simulink model "CustArch_v20"  (R2020a)
settings: Solver=FixedStepDiscrete  StartTime=0.0  StopTime=840000  RelTol=1e-3
libraries: simulink x84, hdlsllib x53
(part 1 of 2)
settings Model: DataTypeOverride=Off  FPTRunName=FPA_Reference  SimulationMode=accelerator  PauseTimes=5600  PacingRate=40  Creator=BuccelliLab  LastModifiedBy=diflo
settings SolverCC: AutoInsertRateTranBlk=on  MinimalZcImpactIntegration=on
settings DataIOCC: LimitDataPoints=on  SaveOutput=off  SaveTime=off  ReturnWorkspaceOutputs=off
settings OptimizationCC: BlockReduction=off  ConditionallyExecuteInputs=off  DefaultParameterBehavior=Inlined  LifeSpan=inf
settings DebuggingCC: SignalRangeChecking=warning  ReadBeforeWriteMsg=DisableAll  WriteAfterWriteMsg=DisableAll  WriteAfterReadMsg=DisableAll  AlgebraicLoopMsg=error  MultiTaskDSMMsg=none  SingleTaskRateTransMsg=error  ParameterDowncastMsg=warning  ParameterOverflowMsg=warning  AllowSymbolicDim=off  StrictBusMsg=ErrorOnBusTreatedAsVector  SFUnexpectedBacktrackingDiag=warning  SFNoUnconditionalDefaultTransitionDiag=warning  SFExecutionAtInitializationDiag=none  ArithmeticOperatorsInVariantConditions=warning
settings HardwareCC: ProdBitPerPointer=32  ProdBitPerSizeT=32  ProdBitPerPtrDiffT=32  ProdLargestAtomicFloat=None  ProdIntDivRoundTo=Undefined  ProdEndianess=Unspecified  ProdWordSize=32  ProdHWDeviceType=ASIC/FPGA->ASIC/FPGA  TargetBitPerPointer=64  TargetBitPerSizeT=64  TargetBitPerPtrDiffT=64  TargetLongLongMode=on  TargetIntDivRoundTo=Zero  TargetEndianess=LittleEndian  TargetWordSize=64  TargetHWDeviceType=Custom Processor->MATLAB Host Computer  ProdEqTarget=off
settings ModelReferenceCC: UpdateModelReferenceTargets=IfOutOfDate
settings SFSimCC: SFSimEcho=off  SimUseLocalCustomCode=off  CustomCodeUndefinedFunction=UseInterfaceOnly
settings RTWCC: RTWUseLocalCustomCode=off
settings CodeAppCC: StateflowObjectComments=on
settings GRTTargetCC: TargetLangStandard=C89/C90 (ANSI)
settings ConfigComp: CovScope=ReferencedModels  CovMetricSettings=dw  CovHtmlReporting=on  CovSaveCumulativeToWorkspaceVar=on  CovSaveSingleToWorkspaceVar=on  CovExternalEMLEnable=off  CovSFcnEnable=off

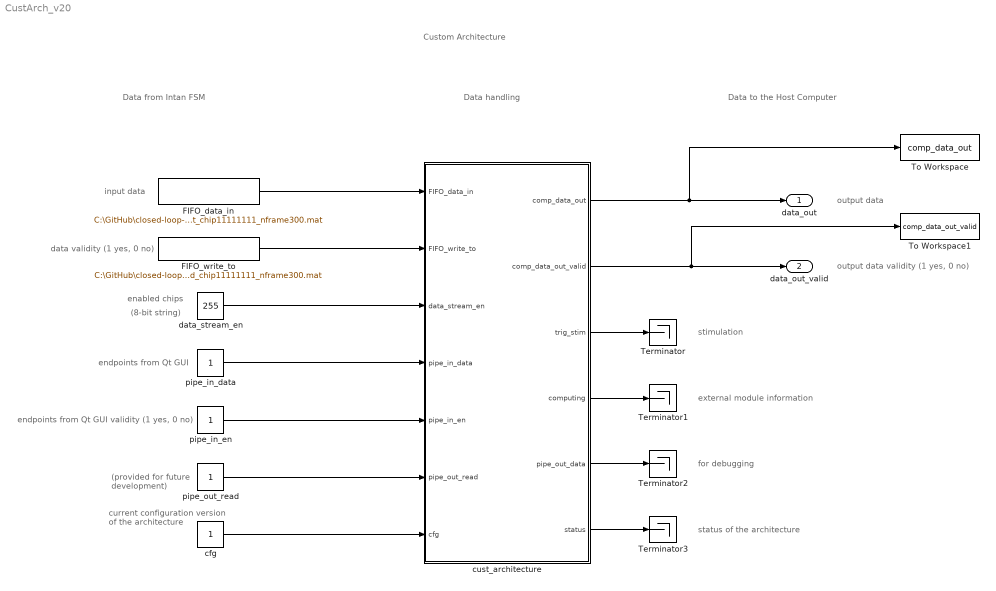
== system CustArch_v20 ==
  note: Data handling
  note: Custom Architecture
  note: output data validity (1 yes, 0 no)
  note: endpoints from Qt GUI
  note: (8-bit string)
  note: enabled chips
  note: data validity (1 yes, 0 no)
  note: input data
  note: endpoints from Qt GUI validity (1 yes, 0 no)
  note: (provided for future
      | development)
  note: current configuration
      | version of the
      | architecture
  note: output data
  note: Data to the Host Computer
  note: stimulation
  note: external module information
  note: for debugging
  note: status of the architecture
  note: Data from Intan FSM
  FIFO_data_in : FromFile  FileName=C:\GitHub\closed-loop-neuroscience\Mattia\Custom_architecture\CustArch_debug\In_Out_Simulink\In\invivo_fsm_out_chip11111111_nframe300.mat  OutDataTypeStr=uint16  SampleTime=1  ExtrapolationBeforeFirstDataPoint=Hold first value  InterpolationWithinTimeRange=Zero order hold  ExtrapolationAfterLastDataPoint=Hold last value
  FIFO_write_to : FromFile  FileName=C:\GitHub\closed-loop-neuroscience\Mattia\Custom_architecture\CustArch_debug\In_Out_Simulink\In\invivo_fsm_valid_chip11111111_nframe300.mat  OutDataTypeStr=boolean  SampleTime=1
  Terminator{,1..3} (4 alike) : Terminator
  To Workspace : ToWorkspace  VariableName=comp_data_out  SaveFormat=Timeseries  SampleTime=-1
  To Workspace1 : ToWorkspace  VariableName=comp_data_out_valid  SaveFormat=Timeseries  SampleTime=-1
  cfg : Constant  OutDataTypeStr=uint16  SampleTime=-1
  cust_architecture : Subsystem
  data_stream_en : Constant  Value=255  OutDataTypeStr=uint8  SampleTime=-1
  pipe_in_data : Constant  OutDataTypeStr=uint16  SampleTime=-1
  pipe_in_en : Constant  OutDataTypeStr=boolean  SampleTime=-1
  pipe_out_read : Constant  OutDataTypeStr=boolean  SampleTime=-1
  data_out : Outport  VectorParamsAs1DForOutWhenUnconnected=off
  data_out_valid : Outport  Port=2  VectorParamsAs1DForOutWhenUnconnected=off
  wires:
  FIFO_data_in/1 -> cust_architecture/1(FIFO_data_in)
  FIFO_write_to/1 -> cust_architecture/2(FIFO_write_to)
  cust_architecture/1(comp_data_out) -> To Workspace/1, data_out/1
  cust_architecture/2(comp_data_out_valid) -> To Workspace1/1, data_out_valid/1
  data_stream_en/1 -> cust_architecture/3(data_stream_en)
  pipe_in_data/1 -> cust_architecture/4(pipe_in_data)
  pipe_in_en/1 -> cust_architecture/5(pipe_in_en)
  pipe_out_read/1 -> cust_architecture/6(pipe_out_read)
  cfg/1 -> cust_architecture/7(cfg)
  cust_architecture/3(trig_stim) -> Terminator/1
  cust_architecture/4(computing) -> Terminator1/1
  cust_architecture/5(pipe_out_data) -> Terminator2/1
  cust_architecture/6(status) -> Terminator3/1

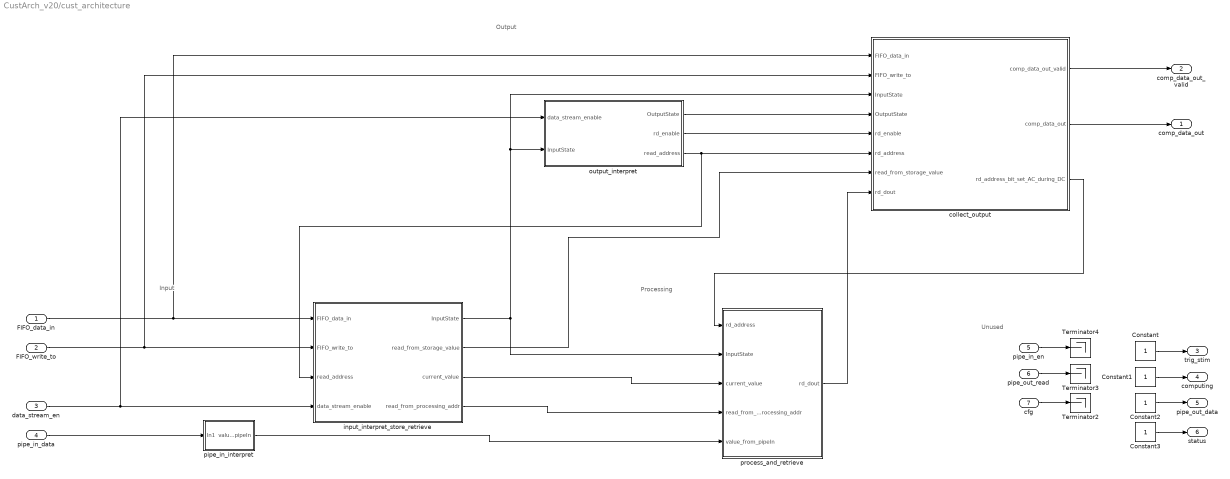
== system CustArch_v20/cust_architecture ==
  note: Unused
  note: Processing
  note: Output
  note: Input
  FIFO_data_in : Inport
  FIFO_write_to : Inport  Port=2
  data_stream_en : Inport  Port=3
  pipe_in_data : Inport  Port=4
  pipe_in_en : Inport  Port=5
  pipe_out_read : Inport  Port=6
  cfg : Inport  Port=7
  Constant : Constant  OutDataTypeStr=uint8  SampleTime=-1
  Constant1 : Constant  OutDataTypeStr=boolean  SampleTime=-1
  Constant2 : Constant  OutDataTypeStr=uint16  SampleTime=-1
  Constant3 : Constant  OutDataTypeStr=uint16  SampleTime=-1
  Terminator2 : Terminator
  Terminator3 : Terminator
  Terminator4 : Terminator
  collect_output : Subsystem
  input_interpret_store_retrieve : Subsystem
  output_interpret : Subsystem
  pipe_in_interpret : Subsystem
  process_and_retrieve : Subsystem
  comp_data_out : Outport  VectorParamsAs1DForOutWhenUnconnected=off
  comp_data_out_valid : Outport  Port=2  OutDataTypeStr=boolean  VectorParamsAs1DForOutWhenUnconnected=off
  trig_stim : Outport  Port=3  VectorParamsAs1DForOutWhenUnconnected=off
  computing : Outport  Port=4  VectorParamsAs1DForOutWhenUnconnected=off
  pipe_out_data : Outport  Port=5  VectorParamsAs1DForOutWhenUnconnected=off
  status : Outport  Port=6  VectorParamsAs1DForOutWhenUnconnected=off
  wires:
  FIFO_data_in/1 -> input_interpret_store_retrieve/1(FIFO_data_in), collect_output/1(FIFO_data_in)
  FIFO_write_to/1 -> collect_output/2(FIFO_write_to), input_interpret_store_retrieve/2(FIFO_write_to)
  data_stream_en/1 -> output_interpret/1(data_stream_enable), input_interpret_store_retrieve/4(data_stream_enable)
  Constant/1 -> trig_stim/1
  Constant1/1 -> computing/1
  Constant2/1 -> pipe_out_data/1
  Constant3/1 -> status/1
  cfg/1 -> Terminator2/1
  pipe_out_read/1 -> Terminator3/1
  pipe_in_en/1 -> Terminator4/1
  collect_output/1(comp_data_out_valid) -> comp_data_out_valid/1
  collect_output/2(comp_data_out) -> comp_data_out/1
  input_interpret_store_retrieve/1(InputState) -> process_and_retrieve/2(InputState), collect_output/3(InputState), output_interpret/2(InputState)
  input_interpret_store_retrieve/2(read_from_storage_value) -> collect_output/7(read_from_storage_value)
  output_interpret/3(read_address) -> collect_output/6(rd_address), input_interpret_store_retrieve/3(read_address)
  output_interpret/1(OutputState) -> collect_output/4(OutputState)
  output_interpret/2(rd_enable) -> collect_output/5(rd_enable)
  pipe_in_data/1 -> pipe_in_interpret/1(In1)
  collect_output/3(rd_address_bit_set_AC_during_DC) -> process_and_retrieve/1(rd_address)
  input_interpret_store_retrieve/3(current_value) -> process_and_retrieve/3(current_value)
  input_interpret_store_retrieve/4(read_from_processing_addr) -> process_and_retrieve/4(read_from_processing_addr)
  pipe_in_interpret/1(value_from_pipeIn) -> process_and_retrieve/5(value_from_pipeIn)
  process_and_retrieve/1(rd_dout) -> collect_output/8(rd_dout)

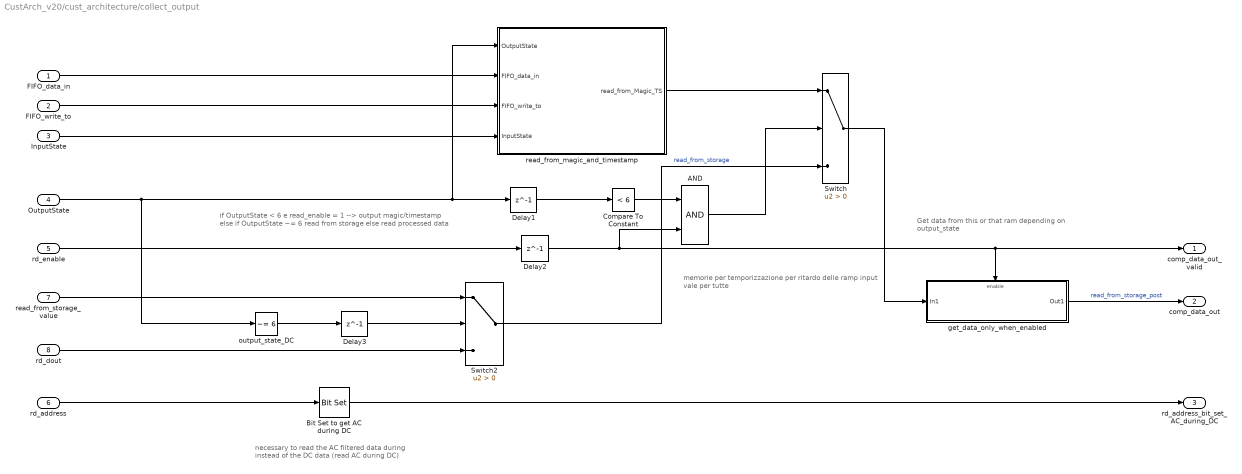
== system CustArch_v20/cust_architecture/collect_output ==
  note: necessary to read the AC filtered data during
      | instead of the DC data (read AC during DC)
  note: if OutputState < 6 e read_enable = 1 --> output magic/timestamp
      | else if OutputState ~= 6 read from storage
      | else read processed data
  note: memorie per temporizzazione per ritardo delle ramp input
      | vale per tutte
  note: Get data from this or that ram depending on output_state
  FIFO_data_in : Inport
  FIFO_write_to : Inport  Port=2
  InputState : Inport  Port=3
  OutputState : Inport  Port=4
  rd_enable : Inport  Port=5
  rd_address : Inport  Port=6
  read_from_storage_value : Inport  Port=7
  rd_dout : Inport  Port=8
  AND : Logic  IconShape=distinctive  AllPortsSameDT=off  OutDataTypeStr=boolean
  Bit Set to get AC during DC : simulink/Logic and Bit Operations/Bit Set  iBit=0
      settings: SourceProductBaseCode=SL
  Compare To Constant : simulink/Logic and Bit Operations/Compare To Constant  relop=<  const=6  OutDataTypeStr=boolean
  Delay1 : Delay  DelayLength=1  InitialCondition=0
  Delay2 : Delay  DelayLength=1  InitialCondition=0
  Delay3 : Delay  DelayLength=1  InitialCondition=0
  Switch : Switch  Criteria=u2 > Threshold
  Switch2 : Switch  Criteria=u2 > Threshold
  get_data_only_when_enabled : Subsystem  TreatAsAtomicUnit=on
  output_state_DC : simulink/Logic and Bit Operations/Compare To Constant  relop=~=  const=6  OutDataTypeStr=boolean
  read_from_magic_and_timestamp : Subsystem
  comp_data_out_valid : Outport
  comp_data_out : Outport  Port=2
  rd_address_bit_set_AC_during_DC : Outport  Port=3
  wires:
  get_data_only_when_enabled/1(Out1) -> comp_data_out/1  "read_from_storage_post"
  FIFO_data_in/1 -> read_from_magic_and_timestamp/2(FIFO_data_in)
  read_from_storage_value/1 -> Switch2/1
  rd_address/1 -> Bit Set to get AC during DC/1
  Delay1/1 -> Compare To Constant/1
  Delay2/1 -> AND/2, comp_data_out_valid/1, get_data_only_when_enabled/Enable
  Switch/1 -> get_data_only_when_enabled/1(In1)
  AND/1 -> Switch/2
  Switch2/1 -> Switch/3  "read_from_storage"
  output_state_DC/1 -> Delay3/1
  Compare To Constant/1 -> AND/1
  Delay3/1 -> Switch2/2
  read_from_magic_and_timestamp/1(read_from_Magic_TS) -> Switch/1
  OutputState/1 -> output_state_DC/1, Delay1/1, read_from_magic_and_timestamp/1(OutputState)
  Bit Set to get AC during DC/1 -> rd_address_bit_set_AC_during_DC/1
  rd_dout/1 -> Switch2/3
  rd_enable/1 -> Delay2/1
  FIFO_write_to/1 -> read_from_magic_and_timestamp/3(FIFO_write_to)
  InputState/1 -> read_from_magic_and_timestamp/4(InputState)

== system CustArch_v20/cust_architecture/input_interpret_store_retrieve ==
  note: data sent to Output
  note: data sent for processing
  note: address sent for processing
  note: reading address
      | from output
  FIFO_data_in : Inport
  FIFO_write_to : Inport  Port=2
  read_address : Inport  Port=3
  data_stream_enable : Inport  Port=4
  InputStateMachine : Stateflow chart  TreatAsAtomicUnit=on
  Interpret_to_RAM_input : Subsystem
  store_and_retrieve_input : Subsystem
  InputState : Outport
  read_from_storage_value : Outport  Port=2
  current_value : Outport  Port=3
  read_from_processing_addr : Outport  Port=4
  wires:
  Interpret_to_RAM_input/4(write address) -> store_and_retrieve_input/3(wr_address)
  Interpret_to_RAM_input/5(wr_en) -> store_and_retrieve_input/4(wr_en)
  InputStateMachine/1(InputState) -> store_and_retrieve_input/5(InputState), InputState/1, Interpret_to_RAM_input/3(InputState)  "InputState"
  store_and_retrieve_input/1(read_from_storage_value) -> read_from_storage_value/1
  Interpret_to_RAM_input/2(inc_source_device) -> InputStateMachine/4(inc_source_device_MSB)
  Interpret_to_RAM_input/1(device_output) -> InputStateMachine/3(channel_0_19)
  Interpret_to_RAM_input/3(wr_din) -> store_and_retrieve_input/2(wr_din)
  FIFO_data_in/1 -> InputStateMachine/1(FIFO_data_in), Interpret_to_RAM_input/1(FIFO_data_in)
  FIFO_write_to/1 -> Interpret_to_RAM_input/2(FIFO_write_to), InputStateMachine/2(FIFO_write_to)
  read_address/1 -> store_and_retrieve_input/1(read address)
  data_stream_enable/1 -> Interpret_to_RAM_input/4(data_stream_enable)
  store_and_retrieve_input/3(read_from_porcessing_addr) -> read_from_processing_addr/1
  store_and_retrieve_input/2(current_value) -> current_value/1

== system CustArch_v20/cust_architecture/output_interpret ==
  note: if InputState == 8 I have processed all the 20 channels (16ch + 4aux)
      | and I start with the output encoding
  data_stream_enable : Inport
  InputState : Inport  Port=2
  Interpret_to_RAM_output : Subsystem
  OutputStateMachine : Stateflow chart  TreatAsAtomicUnit=on
  OutputState : Outport
  rd_enable : Outport  Port=2
  read_address : Outport  Port=3
  wires:
  OutputStateMachine/1(OutputState) -> OutputState/1, Interpret_to_RAM_output/1(OutputState)  "OutputState"
  Interpret_to_RAM_output/1(rd_enable) -> rd_enable/1
  data_stream_enable/1 -> Interpret_to_RAM_output/2(data_stream_en)
  InputState/1 -> OutputStateMachine/1(input_state)
  Interpret_to_RAM_output/2(read address) -> read_address/1

== system CustArch_v20/cust_architecture/pipe_in_interpret ==
  In1 : Inport
  Bit Slice1 : hdlsllib/Logic and Bit Operations/Bit Slice  lidx=15  ridx=8
      settings: SourceProductBaseCode=SL
  Compare To Constant1 : simulink/Logic and Bit Operations/Compare To Constant  relop===  const=2  OutDataTypeStr=boolean
  Constant4 : Constant  Value=5  OutDataTypeStr=uint16  SampleTime=-1
  Memory6 : Memory  InheritSampleTime=on
  Switch1 : Switch  Criteria=u2 > Threshold
  value_from_pipeIn : Outport
  wires:
  Bit Slice1/1 -> Compare To Constant1/1
  Memory6/1 -> Bit Slice1/1
  Compare To Constant1/1 -> Switch1/2
  Switch1/1 -> value_from_pipeIn/1
  Constant4/1 -> Switch1/3
  In1/1 -> Switch1/1, Memory6/1

== system CustArch_v20/cust_architecture/process_and_retrieve ==
  note: The dual-port RAM in the input interpret subsystem introduces
      | a sample of delay. Furthermore, I need one sample more of delay
      | due to the IIR filter --> overall delay of two samples
  note: generally, all sample in the processing subsystem
      | are delayed by two samples --> the memories are
      | needed for this reason
  note: note that these RAM are too big.. I just need 160 and thus a reduced address port width
  note: rd_address from Output
  note: data sent for processing
  note: address sent for processing
  rd_address : Inport
  InputState : Inport  Port=2
  current_value : Inport  Port=3
  read_from_processing_addr : Inport  Port=4
  value_from_pipeIn : Inport  Port=5
  ProcessedData_storage : hdlsllib/HDL RAMs/Dual Port RAM  ram_size=9
      settings: SourceProductBaseCode=SL
  Terminator1 : Terminator
  Terminator7 : Terminator
  filtering : Subsystem
  rd_dout : Outport
  wires:
  ProcessedData_storage/2 -> rd_dout/1
  rd_address/1 -> ProcessedData_storage/4
  ProcessedData_storage/1 -> Terminator7/1
  value_from_pipeIn/1 -> Terminator1/1
  current_value/1 -> filtering/1(current_sample)
  InputState/1 -> filtering/2(In2)
  read_from_processing_addr/1 -> filtering/3(In3)
  filtering/1(filter_output) -> ProcessedData_storage/1
  filtering/2(Out2) -> ProcessedData_storage/2
  filtering/3(Out3) -> ProcessedData_storage/3

== system CustArch_v20/cust_architecture/collect_output/get_data_only_when_enabled ==
  In1 : Inport
  Enable : EnablePort
  Out1 : Outport  InitialOutput=0  VectorParamsAs1DForOutWhenUnconnected=off
  wires:
  In1/1 -> Out1/1

== system CustArch_v20/cust_architecture/collect_output/read_from_magic_and_timestamp ==
  note: This subsystem in needed for save in a specific RAM the magic number
      | and the timestamp
  OutputState : Inport
  FIFO_data_in : Inport  Port=2
  FIFO_write_to : Inport  Port=3
  InputState : Inport  Port=4
  Terminator1 : Terminator
  getting address and enable for Magic and Timestamps : Subsystem
  input_RAM_for_MagicNumber_TimeStamps : hdlsllib/HDL RAMs/Dual Port RAM  ram_size=8
      settings: SourceProductBaseCode=SL
  read_from_Magic_TS : Outport
  wires:
  FIFO_data_in/1 -> input_RAM_for_MagicNumber_TimeStamps/1
  getting address and enable for Magic and Timestamps/2(wr_enable) -> input_RAM_for_MagicNumber_TimeStamps/3
  input_RAM_for_MagicNumber_TimeStamps/2 -> read_from_Magic_TS/1  "read_from_Magic_TS"
  getting address and enable for Magic and Timestamps/1(wr_address) -> input_RAM_for_MagicNumber_TimeStamps/2
  input_RAM_for_MagicNumber_TimeStamps/1 -> Terminator1/1
  OutputState/1 -> input_RAM_for_MagicNumber_TimeStamps/4
  InputState/1 -> getting address and enable for Magic and Timestamps/1(InputState)
  FIFO_write_to/1 -> getting address and enable for Magic and Timestamps/2(FIFO_write_to)

== system CustArch_v20/cust_architecture/input_interpret_store_retrieve/Interpret_to_RAM_input ==
  note: These subsystems identify the sources of the incoming data (amplifier --> source_device and channel number) and
      | determine the address to be associated to the current data for the RAM storage. This statement is valid for all the kind of
      | data except for the magic number and the timestamp that are directly sent to a different RAM in the Output section
  FIFO_data_in : Inport
  FIFO_write_to : Inport  Port=2
  InputState : Inport  Port=3
  data_stream_enable : Inport  Port=4
  RAM address definition : Subsystem
  interpret incoming data : Subsystem
  device_output : Outport
  inc_source_device : Outport  Port=2
  wr_din : Outport  Port=3
  write address : Outport  Port=4
  wr_en : Outport  Port=5
  wires:
  interpret incoming data/4(source_channel_0_159) -> RAM address definition/3(source_channel_0_159)
  interpret incoming data/2(inc_source_device) -> inc_source_device/1
  interpret incoming data/1(source_device) -> RAM address definition/4(source_device)
  data_stream_enable/1 -> interpret incoming data/3(data_stream_enable)
  RAM address definition/3(write_enable_6to15) -> wr_en/1  "wr_en"
  interpret incoming data/3(device_output) -> device_output/1
  InputState/1 -> RAM address definition/2(InputState), interpret incoming data/2(InputState)
  interpret incoming data/5(converter_cnt) -> RAM address definition/5(converter_cnt)
  FIFO_write_to/1 -> RAM address definition/6(write_to), interpret incoming data/1(FIFO_write_to)
  FIFO_data_in/1 -> RAM address definition/1(DataIn)
  RAM address definition/2(wr_addr) -> write address/1  "write address"
  RAM address definition/1(wr_din) -> wr_din/1  "wr_din"

== system CustArch_v20/cust_architecture/input_interpret_store_retrieve/store_and_retrieve_input ==
  note: Two dual-port RAM for storage and processing
  note: current data
  note: data sent to Output
  note: data sent for processing
  note: this memory is for synchronizing the current value and
      | the read_from_porcessing_addr since to ouput a value
      | the dual port RAM needs a single clock
  note: current data
  note: reading address
      | from output
  note: address sent for processing
  note: writing address
  read address : Inport
  wr_din : Inport  Port=2
  wr_address : Inport  Port=3
  wr_en : Inport  Port=4
  InputState : Inport  Port=5
  Compare To Constant : simulink/Logic and Bit Operations/Compare To Constant  relop===  const=7  OutDataTypeStr=boolean
  Delay1 : Delay  DelayLength=1  InitialCondition=0
  Terminator : Terminator
  Terminator6 : Terminator
  input_storage : hdlsllib/HDL RAMs/Dual Port RAM  ram_size=9
      settings: SourceProductBaseCode=SL
  input_storage_for_processing : hdlsllib/HDL RAMs/Dual Port RAM  ram_size=9
      settings: SourceProductBaseCode=SL
  read_from_storage_value : Outport
  current_value : Outport  Port=2
  read_from_porcessing_addr : Outport  Port=3
  wires:
  wr_en/1 -> input_storage/3
  InputState/1 -> Compare To Constant/1
  Compare To Constant/1 -> input_storage_for_processing/3
  input_storage_for_processing/2 -> current_value/1  "current value"
  Delay1/1 -> read_from_porcessing_addr/1, input_storage_for_processing/4  "read from porcessing addr"
  input_storage/1 -> Terminator/1
  wr_address/1 -> Delay1/1, input_storage_for_processing/2, input_storage/2
  wr_din/1 -> input_storage_for_processing/1, input_storage/1
  input_storage/2 -> read_from_storage_value/1  "read_from_storage"
  input_storage_for_processing/1 -> Terminator6/1
  read address/1 -> input_storage/4

== system CustArch_v20/cust_architecture/output_interpret/Interpret_to_RAM_output ==
  OutputState : Inport
  data_stream_en : Inport  Port=2
  Output_State_to_RAM_address (to read) : Subsystem
  "get_enabled_timings " : Subsystem  MinMaxOverflowLogging=MinMaxAndOverflow
  rd_enable : Outport
  read address : Outport  Port=2
  wires:
  "get_enabled_timings "/5(converter_cnt) -> Output_State_to_RAM_address (to read)/6(converter_cnt)
  "get_enabled_timings "/4(source_device) -> Output_State_to_RAM_address (to read)/5(source_device)
  Output_State_to_RAM_address (to read)/2(rd_addr) -> read address/1
  "get_enabled_timings "/3(source_device_enabled) -> Output_State_to_RAM_address (to read)/4(source_device_en)
  "get_enabled_timings "/2(source_channel_0_159) -> Output_State_to_RAM_address (to read)/2(source_channel_0_159)
  "get_enabled_timings "/1(source_channel_en) -> Output_State_to_RAM_address (to read)/1(source_channel_en)
  OutputState/1 -> Output_State_to_RAM_address (to read)/3(OutputState), "get_enabled_timings "/1(OutputState)
  data_stream_en/1 -> "get_enabled_timings "/2(data_stream_en)
  Output_State_to_RAM_address (to read)/1(rd_enable) -> rd_enable/1

== system CustArch_v20/cust_architecture/process_and_retrieve/filtering ==
  note: this memory is to guarantee that the input is already stored
  note: Note: If a read operation occurs simultaneously at the same address
      | as a write operation, old data appears at the read output port (rd_dout).
  current_sample : Inport
  In2 : Inport  Port=2
  In3 : Inport  Port=3
  Delay : Delay  DelayLength=1  InitialCondition=0
  Delay1 : Delay  DelayLength=1  InitialCondition=0
  Delay2 : Delay  DelayLength=1  InitialCondition=0
  Delay3 : Delay  DelayLength=4  InitialCondition=0
  Delay4 : Delay  InitialCondition=0
  Delay5 : Delay  InitialCondition=0
  Delay6 : Delay  InitialCondition=0
  Mux : Mux  Inputs=2
  PreviousData1_storage : hdlsllib/HDL RAMs/Dual Port RAM  ram_size=9
      settings: SourceProductBaseCode=SL
  PreviousData2_storage : hdlsllib/HDL RAMs/Dual Port RAM  ram_size=9
      settings: SourceProductBaseCode=SL
  Terminator2 : Terminator
  Terminator8 : Terminator
  input_state_AC : simulink/Logic and Bit Operations/Compare To Constant  relop===  const=7  OutDataTypeStr=boolean
  two_pole_IIR : Subsystem
  filter_output : Outport
  Out2 : Outport  Port=2
  Out3 : Outport  Port=3
  wires:
  In3/1 -> Delay2/1, PreviousData2_storage/4, PreviousData1_storage/4
  PreviousData1_storage/2 -> PreviousData2_storage/1, Mux/1  "previous_sample"
  Delay2/1 -> PreviousData2_storage/2, Delay5/1, Delay3/1  "new_previous_sample"
  current_sample/1 -> two_pole_IIR/1(current_sample)
  Delay3/1 -> Out2/1
  two_pole_IIR/2(new_previous_sample) -> PreviousData1_storage/1  "new_previous_sample"
  Delay1/1 -> Delay6/1, PreviousData2_storage/3  "write en"
  PreviousData1_storage/1 -> Terminator8/1
  Delay6/1 -> Delay4/1, PreviousData1_storage/3
  In2/1 -> Delay/1
  PreviousData2_storage/1 -> Terminator2/1
  Delay/1 -> input_state_AC/1
  PreviousData2_storage/2 -> Mux/2  "previous_sample"
  input_state_AC/1 -> Delay1/1  "read from porcessing"
  Delay5/1 -> PreviousData1_storage/2
  Mux/1 -> two_pole_IIR/2(previous_sample)
  two_pole_IIR/1(filter_output) -> filter_output/1  "filter_output"
  Delay4/1 -> Out3/1

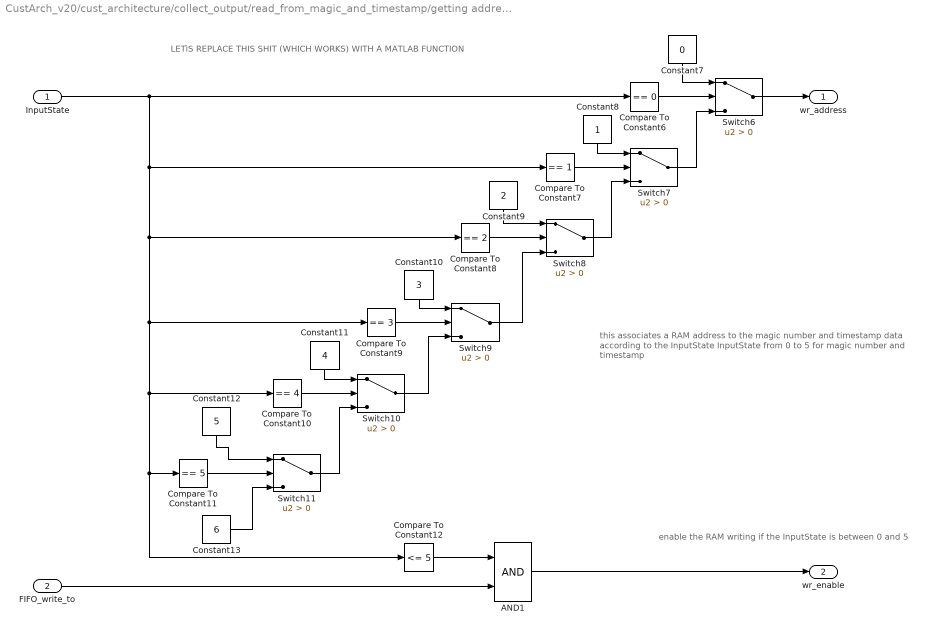
== system CustArch_v20/cust_architecture/collect_output/read_from_magic_and_timestamp/getting address and enable for Magic and Timestamps ==
  note: this associates a RAM address to the magic number and timestamp
      | data according to the InputState
      |
      | InputState from 0 to 5 for magic number and timestamp
  note: LETìS REPLACE THIS SHIT (WHICH WORKS) WITH A MATLAB FUNCTION
  note: enable the RAM writing if the InputState is between 0 and 5
  InputState : Inport
  FIFO_write_to : Inport  Port=2
  AND1 : Logic  IconShape=distinctive  AllPortsSameDT=off  OutDataTypeStr=boolean
  Compare To Constant10 : simulink/Logic and Bit Operations/Compare To Constant  relop===  const=4  OutDataTypeStr=boolean
  Compare To Constant11 : simulink/Logic and Bit Operations/Compare To Constant  relop===  const=5  OutDataTypeStr=boolean
  Compare To Constant12 : simulink/Logic and Bit Operations/Compare To Constant  relop=<=  const=5  OutDataTypeStr=boolean
  Compare To Constant6 : simulink/Logic and Bit Operations/Compare To Constant  relop===  const=0  OutDataTypeStr=boolean
  Compare To Constant7 : simulink/Logic and Bit Operations/Compare To Constant  relop===  const=1  OutDataTypeStr=boolean
  Compare To Constant8 : simulink/Logic and Bit Operations/Compare To Constant  relop===  const=2  OutDataTypeStr=boolean
  Compare To Constant9 : simulink/Logic and Bit Operations/Compare To Constant  relop===  const=3  OutDataTypeStr=boolean
  Constant10 : Constant  Value=3  OutDataTypeStr=uint8  SampleTime=-1
  Constant11 : Constant  Value=4  OutDataTypeStr=uint8  SampleTime=-1
  Constant12 : Constant  Value=5  OutDataTypeStr=uint8  SampleTime=-1
  Constant13 : Constant  Value=6  OutDataTypeStr=uint8  SampleTime=-1
  Constant7 : Constant  Value=0  OutDataTypeStr=uint8  SampleTime=-1
  Constant8 : Constant  OutDataTypeStr=uint8  SampleTime=-1
  Constant9 : Constant  Value=2  OutDataTypeStr=uint8  SampleTime=-1
  Switch{6..11} (6 alike) : Switch  Criteria=u2 > Threshold
  wr_address : Outport  VectorParamsAs1DForOutWhenUnconnected=off
  wr_enable : Outport  Port=2  VectorParamsAs1DForOutWhenUnconnected=off
  wires:
  Constant10/1 -> Switch9/1
  Compare To Constant8/1 -> Switch8/2
  Compare To Constant7/1 -> Switch7/2
  AND1/1 -> wr_enable/1
  Compare To Constant9/1 -> Switch9/2
  Switch10/1 -> Switch9/3
  Compare To Constant12/1 -> AND1/1
  Constant9/1 -> Switch8/1
  Compare To Constant6/1 -> Switch6/2
  FIFO_write_to/1 -> AND1/2
  InputState/1 -> Compare To Constant10/1, Compare To Constant12/1, Compare To Constant11/1, Compare To Constant9/1, Compare To Constant8/1, Compare To Constant7/1, Compare To Constant6/1
  Switch11/1 -> Switch10/3
  Constant11/1 -> Switch10/1
  Switch6/1 -> wr_address/1
  Constant7/1 -> Switch6/1
  Compare To Constant11/1 -> Switch11/2
  Constant12/1 -> Switch11/1
  Constant8/1 -> Switch7/1
  Switch8/1 -> Switch7/3
  Constant13/1 -> Switch11/3
  Switch7/1 -> Switch6/3
  Compare To Constant10/1 -> Switch10/2
  Switch9/1 -> Switch8/3

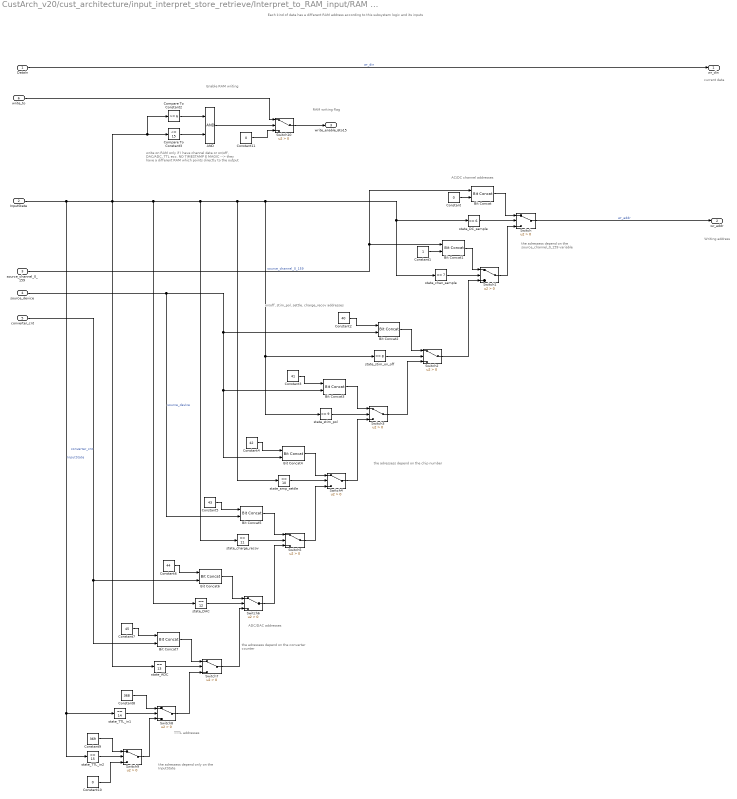
== system CustArch_v20/cust_architecture/input_interpret_store_retrieve/Interpret_to_RAM_input/RAM address definition ==
  note: the adressess depend on the chip number
  note: Each kind of data has a different RAM
      | address according to this subsystem logic
      | and its inputs
  note: AC/DC channel addresses
  note: Writing address
  note: current data
  note: RAM writing flag
  note: write on RAM only if I have channel data or on/off,
      | DAC/ADC, TTL ecc.
      | NO TIMESTAMP E MAGIC --> they have a different
      | RAM which points directly to the output
  note: on/off, stim_pol, settle, charge_recov addresses
  note: ADC/DAC addresses
  note: TTTL addresses
  note: the adressess depend on the converter
      | counter
  note: the adressess depend only on the
      | InputState
  note: the adressess depend on the
      | source_channel_0_159 variable
  note: Enable RAM writing
  DataIn : Inport
  InputState : Inport  Port=2
  source_channel_0_159 : Inport  Port=3
  source_device : Inport  Port=4
  converter_cnt : Inport  Port=5
  write_to : Inport  Port=6  OutDataTypeStr=boolean
  AND : Logic  IconShape=distinctive  AllPortsSameDT=off  OutDataTypeStr=boolean
  Bit Concat{,1..7} (8 alike) : hdlsllib/Logic and Bit Operations/Bit Concat  numInputs=2
  Compare To Constant2 : simulink/Logic and Bit Operations/Compare To Constant  relop=>=  const=6  OutDataTypeStr=boolean
  Compare To Constant3 : simulink/Logic and Bit Operations/Compare To Constant  relop=<=  const=15  OutDataTypeStr=boolean
  Constant : Constant  Value=0  OutDataTypeStr=boolean  SampleTime=-1
  Constant1 : Constant  OutDataTypeStr=boolean  SampleTime=-1
  Constant10 : Constant  Value=0  OutDataTypeStr=fixdt(0,9)  SampleTime=-1
  Constant11 : Constant  Value=0  OutDataTypeStr=boolean  SampleTime=-1
  Constant2 : Constant  Value=40  OutDataTypeStr=fixdt(0,6)  SampleTime=-1
  Constant3 : Constant  Value=41  OutDataTypeStr=fixdt(0,6)  SampleTime=-1
  Constant4 : Constant  Value=42  OutDataTypeStr=fixdt(0,6)  SampleTime=-1
  Constant5 : Constant  Value=43  OutDataTypeStr=fixdt(0,6)  SampleTime=-1
  Constant6 : Constant  Value=44  OutDataTypeStr=fixdt(0,6)  SampleTime=-1
  Constant7 : Constant  Value=45  OutDataTypeStr=fixdt(0,6)  SampleTime=-1
  Constant8 : Constant  Value=368  OutDataTypeStr=fixdt(0,9)  SampleTime=-1
  Constant9 : Constant  Value=369  OutDataTypeStr=fixdt(0,9)  SampleTime=-1
  Switch{,1..10} (11 alike) : Switch  Criteria=u2 > Threshold
  state_ADC : simulink/Logic and Bit Operations/Compare To Constant  relop===  const=13  OutDataTypeStr=boolean
  state_DAC : simulink/Logic and Bit Operations/Compare To Constant  relop===  const=12  OutDataTypeStr=boolean
  state_DC_sample : simulink/Logic and Bit Operations/Compare To Constant  relop===  const=6  OutDataTypeStr=boolean
  state_TTL_in1 : simulink/Logic and Bit Operations/Compare To Constant  relop===  const=14  OutDataTypeStr=boolean
  state_TTL_in2 : simulink/Logic and Bit Operations/Compare To Constant  relop===  const=15  OutDataTypeStr=boolean
  state_amp_settle : simulink/Logic and Bit Operations/Compare To Constant  relop===  const=10  OutDataTypeStr=boolean
  state_chan_sample : simulink/Logic and Bit Operations/Compare To Constant  relop===  const=7  OutDataTypeStr=boolean
  state_charge_recov : simulink/Logic and Bit Operations/Compare To Constant  relop===  const=11  OutDataTypeStr=boolean
  state_stim_on_off : simulink/Logic and Bit Operations/Compare To Constant  relop===  const=8  OutDataTypeStr=boolean
  state_stim_pol : simulink/Logic and Bit Operations/Compare To Constant  relop===  const=9  OutDataTypeStr=boolean
  wr_din : Outport  VectorParamsAs1DForOutWhenUnconnected=off
  wr_addr : Outport  Port=2  OutDataTypeStr=fixdt(0,9,0)  VectorParamsAs1DForOutWhenUnconnected=off
  write_enable_6to15 : Outport  Port=3  OutDataTypeStr=boolean  VectorParamsAs1DForOutWhenUnconnected=off
  wires:
  state_DC_sample/1 -> Switch/2
  source_channel_0_159/1 -> Bit Concat1/1, Bit Concat/1  "source_channel_0_159"
  Constant/1 -> Bit Concat/2
  Bit Concat/1 -> Switch/1
  state_chan_sample/1 -> Switch1/2
  Constant1/1 -> Bit Concat1/2
  Bit Concat1/1 -> Switch1/1
  Switch1/1 -> Switch/3
  Switch/1 -> wr_addr/1  "wr_addr"
  Constant2/1 -> Bit Concat2/1
  Bit Concat2/1 -> Switch2/1
  state_stim_on_off/1 -> Switch2/2
  Switch2/1 -> Switch1/3
  Constant3/1 -> Bit Concat3/1
  state_stim_pol/1 -> Switch3/2
  Bit Concat3/1 -> Switch3/1
  Switch3/1 -> Switch2/3
  Constant4/1 -> Bit Concat4/1
  state_amp_settle/1 -> Switch4/2
  Bit Concat4/1 -> Switch4/1
  Switch4/1 -> Switch3/3
  Bit Concat5/1 -> Switch5/1
  state_charge_recov/1 -> Switch5/2
  Constant5/1 -> Bit Concat5/1
  source_device/1 -> Bit Concat5/2, Bit Concat4/2, Bit Concat3/2, Bit Concat2/2  "source_device"
  Switch5/1 -> Switch4/3
  Bit Concat6/1 -> Switch6/1
  state_DAC/1 -> Switch6/2
  Constant6/1 -> Bit Concat6/1
  Switch6/1 -> Switch5/3
  converter_cnt/1 -> Bit Concat7/2, Bit Concat6/2  "converter_cnt"
  Bit Concat7/1 -> Switch7/1
  state_ADC/1 -> Switch7/2
  Constant7/1 -> Bit Concat7/1
  Switch7/1 -> Switch6/3
  state_TTL_in1/1 -> Switch8/2
  Constant8/1 -> Switch8/1
  Switch8/1 -> Switch7/3
  state_TTL_in2/1 -> Switch9/2
  Constant9/1 -> Switch9/1
  Switch9/1 -> Switch8/3
  Constant10/1 -> Switch9/3
  DataIn/1 -> wr_din/1  "wr_din"
  Compare To Constant3/1 -> AND/2
  InputState/1 -> state_TTL_in1/1, state_TTL_in2/1, state_ADC/1, state_DAC/1, state_charge_recov/1, state_amp_settle/1, state_stim_pol/1, state_stim_on_off/1, state_chan_sample/1, state_DC_sample/1, Compare To Constant2/1, Compare To Constant3/1  "InputState"
  AND/1 -> Switch10/2
  Switch10/1 -> write_enable_6to15/1
  write_to/1 -> Switch10/1
  Compare To Constant2/1 -> AND/1
  Constant11/1 -> Switch10/3

== system CustArch_v20/cust_architecture/input_interpret_store_retrieve/Interpret_to_RAM_input/interpret incoming data ==
  note: counter of the converters
  note: to reduce the number of bit to encode
      | the ADC/DAC counter since it could takes
      | values from 0 to 7
  note: check ADC/DAC state
  note: ADC/DAC counter
      | (from 0 to 7 for each)
  note: to reduce the number of bit to encode
      | the soure device since it could takes
      | values from 0 to 7
  note: amplifier chip under
      | processing
  note: channel data
      | address
  note: channel (electrode) under
      | processing
  note: necessary to move
      | forward from state 6 to 8
  FIFO_write_to : Inport
  InputState : Inport  Port=2
  data_stream_enable : Inport  Port=3
  Bit Slice : hdlsllib/Logic and Bit Operations/Bit Slice  lidx=2  ridx=0
      settings: SourceProductBaseCode=SL
  Bit Slice1 : hdlsllib/Logic and Bit Operations/Bit Slice  lidx=2  ridx=0
      settings: SourceProductBaseCode=SL
  HDL Counter : hdlsllib/Sources/HDL Counter  CountType=Count limited  CountInit=0  CountStep=1  CountMax=7  CountFromType=Specify  CountFrom=0  CountResetPort=off  CountLoadPort=off  CountEnbPort=on  CountDirPort=off  CountDataType=Unsigned  CountWordLen=8  CountFracLen=0  CountSampTime=1
  "condition to count DAC or ADC " : Subsystem
  get_sources_and_RAM_addresses : Subsystem
  source_device : Outport  VectorParamsAs1DForOutWhenUnconnected=off
  inc_source_device : Outport  Port=2  VectorParamsAs1DForOutWhenUnconnected=off
  device_output : Outport  Port=3  VectorParamsAs1DForOutWhenUnconnected=off
  source_channel_0_159 : Outport  Port=4  VectorParamsAs1DForOutWhenUnconnected=off
  converter_cnt : Outport  Port=5  VectorParamsAs1DForOutWhenUnconnected=off
  wires:
  FIFO_write_to/1 -> "condition to count DAC or ADC "/1(fifo_write_to), get_sources_and_RAM_addresses/1(FIFO_write_to)
  data_stream_enable/1 -> get_sources_and_RAM_addresses/3(data_stream_enable)
  InputState/1 -> "condition to count DAC or ADC "/2(input_state), get_sources_and_RAM_addresses/2(InputState)
  "condition to count DAC or ADC "/1(Out1) -> HDL Counter/1
  Bit Slice/1 -> converter_cnt/1
  HDL Counter/1 -> Bit Slice/1
  get_sources_and_RAM_addresses/1(source_device) -> Bit Slice1/1
  get_sources_and_RAM_addresses/3(source_channel) -> source_channel_0_159/1
  get_sources_and_RAM_addresses/2(device_output) -> device_output/1
  Bit Slice1/1 -> source_device/1
  get_sources_and_RAM_addresses/4(inc_source_device) -> inc_source_device/1

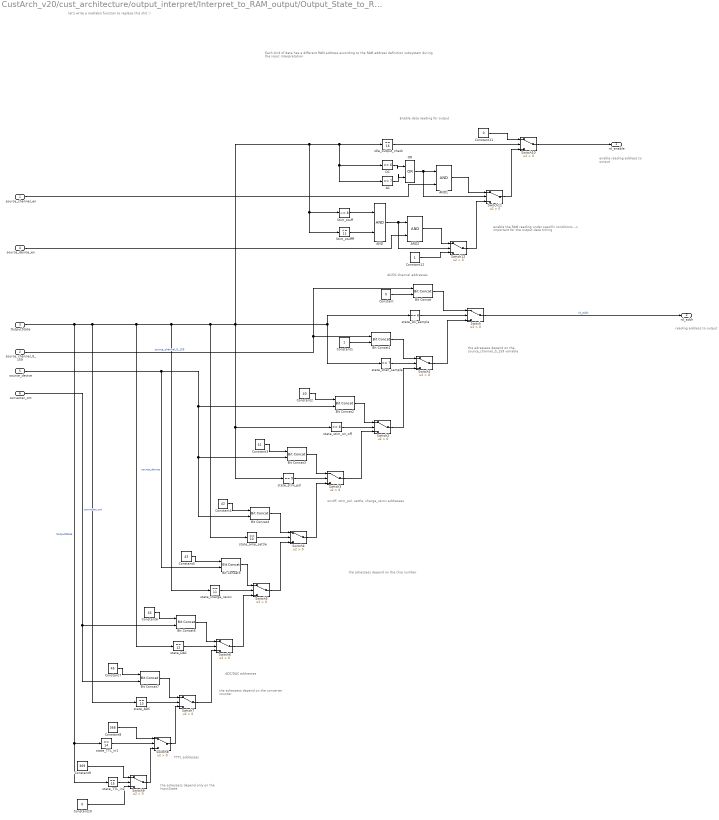
== system CustArch_v20/cust_architecture/output_interpret/Interpret_to_RAM_output/Output_State_to_RAM_address (to read) ==
  note: reading address
      | to output
  note: enable the RAM reading under specific conditions
      | --> important for the output data timing
  note: Enable data reading for output
  note: let's write a matlab/s function to replace this shit :)
  note: TTTL addresses
  note: the adressess depend on the chip number
  note: the adressess depend only on the
      | InputState
  note: the adressess depend on the converter
      | counter
  note: on/off, stim_pol, settle, charge_recov addresses
  note: ADC/DAC addresses
  note: AC/DC channel addresses
  note: the adressess depend on the
      | source_channel_0_159 variable
  note: Each kind of data has a different RAM
      | address according to the
      | RAM address definition subsystem during the
      | input interpretation
  note: enable reading address
      | to output
  source_channel_en : Inport
  source_channel_0_159 : Inport  Port=2
  OutputState : Inport  Port=3
  source_device_en : Inport  Port=4
  source_device : Inport  Port=5
  converter_cnt : Inport  Port=6
  AC : simulink/Logic and Bit Operations/Compare To Constant  relop===  const=7  OutDataTypeStr=boolean
  AND : Logic  IconShape=distinctive  AllPortsSameDT=off  OutDataTypeStr=boolean
  AND1 : Logic  IconShape=distinctive  AllPortsSameDT=off  OutDataTypeStr=boolean
  AND2 : Logic  IconShape=distinctive  AllPortsSameDT=off  OutDataTypeStr=boolean
  Bit Concat{,1..7} (8 alike) : hdlsllib/Logic and Bit Operations/Bit Concat  numInputs=2
  Constant : Constant  Value=0  OutDataTypeStr=boolean  SampleTime=-1
  Constant1 : Constant  OutDataTypeStr=boolean  SampleTime=-1
  Constant10 : Constant  Value=0  OutDataTypeStr=fixdt(0,9)  SampleTime=-1
  Constant11 : Constant  Value=0  OutDataTypeStr=boolean  SampleTime=-1
  Constant12 : Constant  OutDataTypeStr=boolean  SampleTime=-1
  Constant2 : Constant  Value=40  OutDataTypeStr=fixdt(0,6)  SampleTime=-1
  Constant3 : Constant  Value=41  OutDataTypeStr=fixdt(0,6)  SampleTime=-1
  Constant4 : Constant  Value=42  OutDataTypeStr=fixdt(0,6)  SampleTime=-1
  Constant5 : Constant  Value=43  OutDataTypeStr=fixdt(0,6)  SampleTime=-1
  Constant6 : Constant  Value=44  OutDataTypeStr=fixdt(0,6)  SampleTime=-1
  Constant7 : Constant  Value=45  OutDataTypeStr=fixdt(0,6)  SampleTime=-1
  Constant8 : Constant  Value=368  OutDataTypeStr=fixdt(0,9)  SampleTime=-1
  Constant9 : Constant  Value=369  OutDataTypeStr=fixdt(0,9)  SampleTime=-1
  DC : simulink/Logic and Bit Operations/Compare To Constant  relop===  const=6  OutDataTypeStr=boolean
  OR : Logic  Operator=OR  IconShape=distinctive  AllPortsSameDT=off  OutDataTypeStr=boolean
  Stim_stuff : simulink/Logic and Bit Operations/Compare To Constant  relop=>=  const=8  OutDataTypeStr=boolean
  Stim_stuffff : simulink/Logic and Bit Operations/Compare To Constant  relop=<=  const=11  OutDataTypeStr=boolean
  Switch{,1..12} (13 alike) : Switch  Criteria=u2 > Threshold
  idle_output_check : simulink/Logic and Bit Operations/Compare To Constant  relop===  const=16  OutDataTypeStr=boolean
  state_ADC : simulink/Logic and Bit Operations/Compare To Constant  relop===  const=13  OutDataTypeStr=boolean
  state_DAC : simulink/Logic and Bit Operations/Compare To Constant  relop===  const=12  OutDataTypeStr=boolean
  state_DC_sample : simulink/Logic and Bit Operations/Compare To Constant  relop===  const=6  OutDataTypeStr=boolean
  state_TTL_in1 : simulink/Logic and Bit Operations/Compare To Constant  relop===  const=14  OutDataTypeStr=boolean
  state_TTL_in2 : simulink/Logic and Bit Operations/Compare To Constant  relop===  const=15  OutDataTypeStr=boolean
  state_amp_settle : simulink/Logic and Bit Operations/Compare To Constant  relop===  const=10  OutDataTypeStr=boolean
  state_chan_sample : simulink/Logic and Bit Operations/Compare To Constant  relop===  const=7  OutDataTypeStr=boolean
  state_charge_recov : simulink/Logic and Bit Operations/Compare To Constant  relop===  const=11  OutDataTypeStr=boolean
  state_stim_on_off : simulink/Logic and Bit Operations/Compare To Constant  relop===  const=8  OutDataTypeStr=boolean
  state_stim_pol : simulink/Logic and Bit Operations/Compare To Constant  relop===  const=9  OutDataTypeStr=boolean
  rd_enable : Outport  VectorParamsAs1DForOutWhenUnconnected=off
  rd_addr : Outport  Port=2  OutDataTypeStr=fixdt(0,9,0)  VectorParamsAs1DForOutWhenUnconnected=off
  wires:
  state_DC_sample/1 -> Switch/2
  source_channel_0_159/1 -> Bit Concat1/1, Bit Concat/1  "source_channel_0_159"
  Constant/1 -> Bit Concat/2
  Bit Concat/1 -> Switch/1
  state_chan_sample/1 -> Switch1/2
  Constant1/1 -> Bit Concat1/2
  Bit Concat1/1 -> Switch1/1
  Switch1/1 -> Switch/3
  Switch/1 -> rd_addr/1  "rd_addr"
  Constant2/1 -> Bit Concat2/1
  Bit Concat2/1 -> Switch2/1
  state_stim_on_off/1 -> Switch2/2
  Switch2/1 -> Switch1/3
  Constant3/1 -> Bit Concat3/1
  state_stim_pol/1 -> Switch3/2
  Bit Concat3/1 -> Switch3/1
  Switch3/1 -> Switch2/3
  Constant4/1 -> Bit Concat4/1
  state_amp_settle/1 -> Switch4/2
  Bit Concat4/1 -> Switch4/1
  Switch4/1 -> Switch3/3
  Bit Concat5/1 -> Switch5/1
  state_charge_recov/1 -> Switch5/2
  Constant5/1 -> Bit Concat5/1
  source_device/1 -> Bit Concat5/2, Bit Concat4/2, Bit Concat3/2, Bit Concat2/2  "source_device"
  Switch5/1 -> Switch4/3
  Bit Concat6/1 -> Switch6/1
  state_DAC/1 -> Switch6/2
  Constant6/1 -> Bit Concat6/1
  Switch6/1 -> Switch5/3
  converter_cnt/1 -> Bit Concat7/2, Bit Concat6/2  "converter_cnt"
  Bit Concat7/1 -> Switch7/1
  state_ADC/1 -> Switch7/2
  Constant7/1 -> Bit Concat7/1
  Switch7/1 -> Switch6/3
  state_TTL_in1/1 -> Switch8/2
  Constant8/1 -> Switch8/1
  OutputState/1 -> state_TTL_in2/1, state_TTL_in1/1, state_DAC/1, state_amp_settle/1, state_stim_pol/1, state_stim_on_off/1, state_DC_sample/1, state_chan_sample/1, AC/1, DC/1, idle_output_check/1, Stim_stuffff/1, Stim_stuff/1, state_charge_recov/1, state_ADC/1  "OutputState"
  Switch8/1 -> Switch7/3
  state_TTL_in2/1 -> Switch9/2
  Constant9/1 -> Switch9/1
  Switch9/1 -> Switch8/3
  Constant10/1 -> Switch9/3
  DC/1 -> OR/1
  AC/1 -> OR/2
  OR/1 -> Switch11/2, AND1/1
  idle_output_check/1 -> Switch10/2
  Stim_stuff/1 -> AND/1
  Stim_stuffff/1 -> AND/2
  AND/1 -> Switch12/2, AND2/1
  source_channel_en/1 -> AND1/2
  source_device_en/1 -> AND2/2
  Constant11/1 -> Switch10/1
  Switch11/1 -> Switch10/3
  AND1/1 -> Switch11/1
  AND2/1 -> Switch12/1
  Switch12/1 -> Switch11/3
  Constant12/1 -> Switch12/3
  Switch10/1 -> rd_enable/1

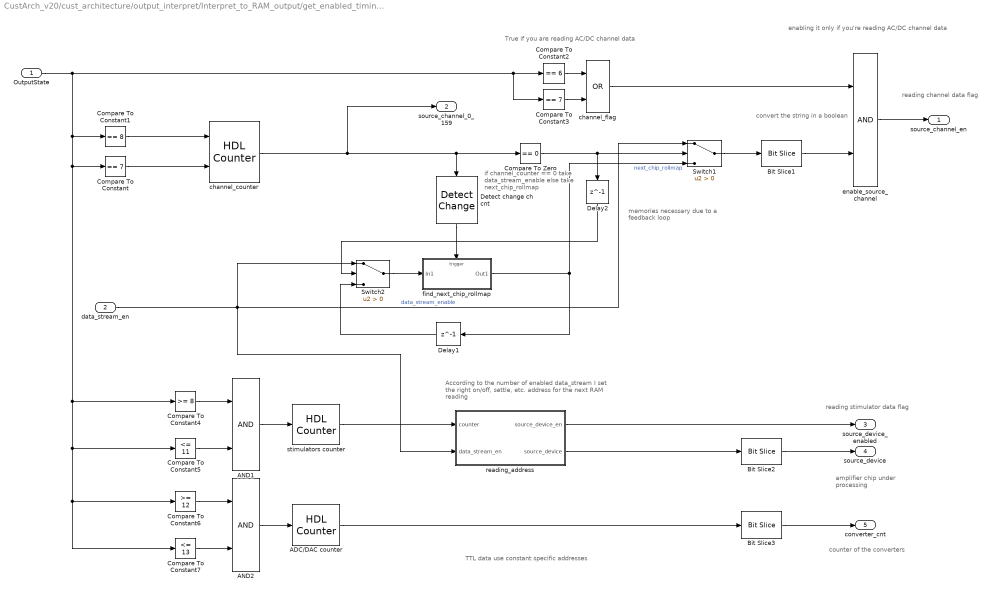
== system CustArch_v20/cust_architecture/output_interpret/Interpret_to_RAM_output/get_enabled_timings  ==
  note: reading channel data flag
  note: memories necessary due to
      | a feedback loop
  note: if channel_counter == 0
      | take data_stream_enable
      | else take next_chip_rollmap
  note: amplifier chip under
      | processing
  note: According to the number of enabled data_stream
      | I set the right on/off, settle, etc. address for the next
      | RAM reading
  note: convert the string
      | in a boolean
  note: True if you are reading AC/DC channel data
  note: enabling it only if you're reading AC/DC channel data
  note: TTL data use constant specific addresses
  note: reading stimulator data flag
  note: counter of the converters
  OutputState : Inport
  data_stream_en : Inport  Port=2
  ADC/DAC counter : hdlsllib/Sources/HDL Counter  CountType=Count limited  CountInit=0  CountStep=1  CountMax=7  CountFromType=Specify  CountFrom=0  CountResetPort=off  CountLoadPort=off  CountEnbPort=on  CountDirPort=off  CountDataType=Unsigned  CountWordLen=8  CountFracLen=0  CountSampTime=1
  AND1 : Logic  IconShape=distinctive  AllPortsSameDT=off  OutDataTypeStr=boolean
  AND2 : Logic  IconShape=distinctive  AllPortsSameDT=off  OutDataTypeStr=boolean
  Bit Slice1 : hdlsllib/Logic and Bit Operations/Bit Slice  lidx=0  ridx=0
      settings: SourceProductBaseCode=SL
  Bit Slice2 : hdlsllib/Logic and Bit Operations/Bit Slice  lidx=2  ridx=0
      settings: SourceProductBaseCode=SL
  Bit Slice3 : hdlsllib/Logic and Bit Operations/Bit Slice  lidx=2  ridx=0
      settings: SourceProductBaseCode=SL
  Compare To Constant : simulink/Logic and Bit Operations/Compare To Constant  relop===  const=7  OutDataTypeStr=boolean
  Compare To Constant1 : simulink/Logic and Bit Operations/Compare To Constant  relop===  const=8  OutDataTypeStr=boolean
  Compare To Constant2 : simulink/Logic and Bit Operations/Compare To Constant  relop===  const=6  OutDataTypeStr=boolean
  Compare To Constant3 : simulink/Logic and Bit Operations/Compare To Constant  relop===  const=7  OutDataTypeStr=boolean
  Compare To Constant4 : simulink/Logic and Bit Operations/Compare To Constant  relop=>=  const=8  OutDataTypeStr=boolean
  Compare To Constant5 : simulink/Logic and Bit Operations/Compare To Constant  relop=<=  const=11  OutDataTypeStr=boolean
  Compare To Constant6 : simulink/Logic and Bit Operations/Compare To Constant  relop=>=  const=12  OutDataTypeStr=boolean
  Compare To Constant7 : simulink/Logic and Bit Operations/Compare To Constant  relop=<=  const=13  OutDataTypeStr=boolean
  Compare To Zero : simulink/Logic and Bit Operations/Compare To Zero  relop===  OutDataTypeStr=boolean
  Delay1 : Delay  DelayLength=1  InitialCondition=0
  Delay2 : Delay  DelayLength=1  InitialCondition=0
  Detect change ch cnt : simulink/Logic and Bit Operations/Detect Change  vinit=0  OutDataTypeStr=boolean
  Switch1 : Switch  Criteria=u2 > Threshold
  Switch2 : Switch  Criteria=u2 > Threshold
  channel_counter : hdlsllib/Sources/HDL Counter  CountType=Count limited  CountInit=0  CountStep=1  CountMax=159  CountFromType=Specify  CountFrom=0  CountResetPort=on  CountLoadPort=off  CountEnbPort=on  CountDirPort=off  CountDataType=Unsigned  CountWordLen=8  CountFracLen=0  CountSampTime=1
  channel_flag : Logic  Operator=OR  IconShape=distinctive  AllPortsSameDT=off  OutDataTypeStr=boolean
  enable_source_channel : Logic  IconShape=distinctive  AllPortsSameDT=off  OutDataTypeStr=boolean
  find_next_chip_rollmap : Subsystem  TreatAsAtomicUnit=on
  reading_address : Subsystem
  stimulators counter : hdlsllib/Sources/HDL Counter  CountType=Count limited  CountInit=0  CountStep=1  CountMax=7  CountFromType=Specify  CountFrom=0  CountResetPort=off  CountLoadPort=off  CountEnbPort=on  CountDirPort=off  CountDataType=Unsigned  CountWordLen=8  CountFracLen=0  CountSampTime=1
  source_channel_en : Outport  VectorParamsAs1DForOutWhenUnconnected=off
  source_channel_0_159 : Outport  Port=2  OutMin=0  OutMax=159  OutDataTypeStr=uint8  VectorParamsAs1DForOutWhenUnconnected=off  LockScale=on
  source_device_enabled : Outport  Port=3  VectorParamsAs1DForOutWhenUnconnected=off
  source_device : Outport  Port=4  VectorParamsAs1DForOutWhenUnconnected=off
  converter_cnt : Outport  Port=5  VectorParamsAs1DForOutWhenUnconnected=off
  wires:
  channel_counter/1 -> Detect change ch cnt/1, Compare To Zero/1, source_channel_0_159/1
  Detect change ch cnt/1 -> find_next_chip_rollmap/Trigger
  find_next_chip_rollmap/1(Out1) -> Delay1/1, Switch1/3  "next_chip_rollmap"
  Delay1/1 -> Switch2/3
  Switch2/1 -> find_next_chip_rollmap/1(In1)
  Compare To Zero/1 -> Delay2/1, Switch1/2
  Delay2/1 -> Switch2/2
  Compare To Constant3/1 -> channel_flag/2
  Compare To Constant2/1 -> channel_flag/1
  channel_flag/1 -> enable_source_channel/1
  enable_source_channel/1 -> source_channel_en/1
  Switch1/1 -> Bit Slice1/1
  Bit Slice1/1 -> enable_source_channel/2
  Compare To Constant4/1 -> AND1/1
  Compare To Constant5/1 -> AND1/2
  reading_address/1(source_device_en) -> source_device_enabled/1
  Bit Slice2/1 -> source_device/1
  AND1/1 -> stimulators counter/1
  stimulators counter/1 -> reading_address/1("counter ")
  reading_address/2(source_device) -> Bit Slice2/1
  data_stream_en/1 -> Switch1/1, reading_address/2(data_stream_en), Switch2/1  "data_stream_enable"
  Compare To Constant6/1 -> AND2/1
  Bit Slice3/1 -> converter_cnt/1
  OutputState/1 -> Compare To Constant1/1, Compare To Constant/1, Compare To Constant6/1, Compare To Constant7/1, Compare To Constant5/1, Compare To Constant4/1, Compare To Constant3/1, Compare To Constant2/1
  Compare To Constant7/1 -> AND2/2
  AND2/1 -> ADC/DAC counter/1
  ADC/DAC counter/1 -> Bit Slice3/1
  Compare To Constant1/1 -> channel_counter/1
  Compare To Constant/1 -> channel_counter/2

== system CustArch_v20/cust_architecture/process_and_retrieve/filtering/two_pole_IIR ==
  current_sample : Inport  OutDataTypeStr=fixdt(0,16,0)
  previous_sample : Inport  Port=2
  Constant : Constant  Value=32768  OutDataTypeStr=fixdt(0,16,0)  SampleTime=-1
  Constant1 : Constant  Value=32768  OutDataTypeStr=fixdt(0,16,0)  SampleTime=-1
  HP_Butter_2nd : Subsystem  Tag=FilterWizardSubSystem
      settings: ErrorFcn=dspFilterRealizedInBasicElemsAlgLoopErrFcnCallback
  Subtract : Sum  Inputs=+-  AccumDataTypeStr=fixdt(1,32,14)  OutDataTypeStr=fixdt(1,32,15)
  Subtract1 : Sum  AccumDataTypeStr=fixdt(1,32,14)  OutDataTypeStr=fixdt(0,16,0)
  filter_output : Outport  InitialOutput=[0]
  new_previous_sample : Outport  Port=2  InitialOutput=[0]
  wires:
  Constant/1 -> Subtract/2
  Subtract/1 -> HP_Butter_2nd/1(Input)
  current_sample/1 -> Subtract/1
  Constant1/1 -> Subtract1/2
  previous_sample/1 -> HP_Butter_2nd/2(previous_samples)
  HP_Butter_2nd/1(Output) -> Subtract1/1
  Subtract1/1 -> filter_output/1
  HP_Butter_2nd/2(Output1) -> new_previous_sample/1

== system CustArch_v20/cust_architecture/input_interpret_store_retrieve/Interpret_to_RAM_input/interpret incoming data/condition to count DAC or ADC  ==
  fifo_write_to : Inport
  input_state : Inport  Port=2
  AND : Logic  IconShape=distinctive  AllPortsSameDT=off  OutDataTypeStr=boolean
  OR : Logic  Operator=OR  IconShape=distinctive  AllPortsSameDT=off  OutDataTypeStr=boolean
  is state_ADC : simulink/Logic and Bit Operations/Compare To Constant  relop===  const=13  OutDataTypeStr=boolean
  is state_DAC : simulink/Logic and Bit Operations/Compare To Constant  relop===  const=12  OutDataTypeStr=boolean
  Out1 : Outport  VectorParamsAs1DForOutWhenUnconnected=off
  wires:
  input_state/1 -> is state_DAC/1, is state_ADC/1
  is state_DAC/1 -> OR/1
  is state_ADC/1 -> OR/2
  fifo_write_to/1 -> AND/1
  OR/1 -> AND/2
  AND/1 -> Out1/1
